simulink model "untitled"  (R2023a)
settings: Solver=VariableStepAuto  StartTime=0.0  StopTime=100  RelTol=1e-3
settings Model: Creator=Sumeadh  LastModifiedBy=Sumeadh

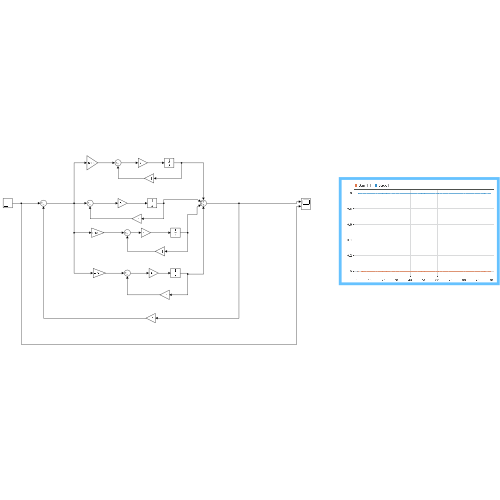
[thumbnail: Simulink's stored preview of the top-level diagram]
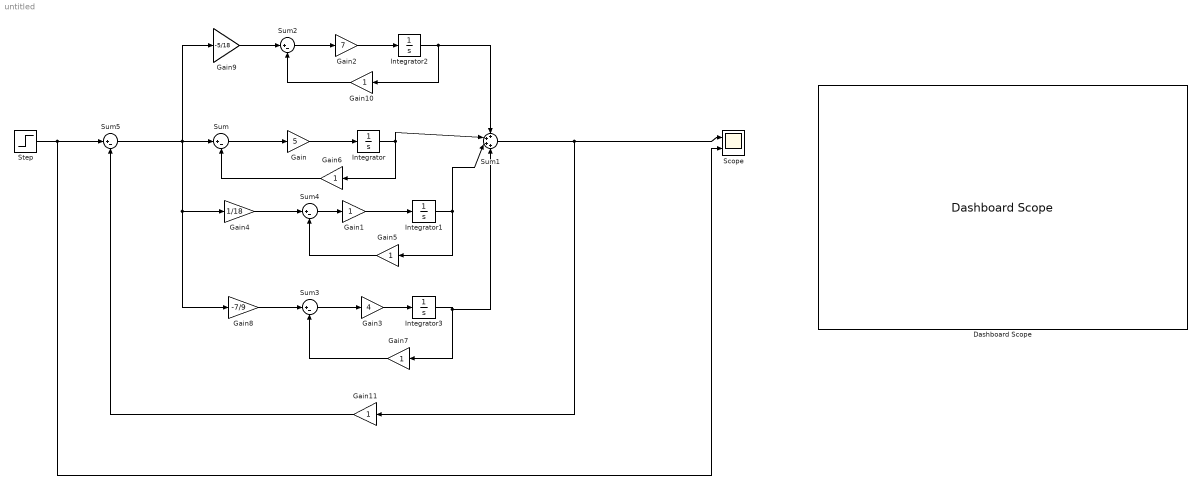
== system untitled ==
  Dashboard Scope : DashboardScope
  Gain : Gain  Gain=5
  Gain{1,5..7,10..11} (6 alike) : Gain
  Gain2 : Gain  Gain=7
  Gain3 : Gain  Gain=4
  Gain4 : Gain  Gain=1/18
  Gain8 : Gain  Gain=-7/9
  Gain9 : Gain  Gain=-5/18
  Integrator{,1..3} (4 alike) : Integrator
  Scope : Scope  NumInputPorts=2
  Step : Step  SampleTime=0
  Sum{,2..5} (5 alike) : Sum  Inputs=|+-
  Sum1 : Sum  Inputs=++++
  wires:
  Sum5/1 -> Gain9/1, Gain4/1, Gain8/1, Sum/1
  Sum/1 -> Gain/1
  Gain/1 -> Integrator/1
  Integrator/1 -> Sum1/2, Gain6/1
  Gain1/1 -> Integrator1/1
  Sum4/1 -> Gain1/1
  Integrator1/1 -> Sum1/3, Gain5/1
  Gain5/1 -> Sum4/2
  Gain4/1 -> Sum4/1
  Gain6/1 -> Sum/2
  Sum1/1 -> Gain11/1, Scope/1
  Gain3/1 -> Integrator3/1
  Integrator3/1 -> Sum1/4, Gain7/1
  Gain7/1 -> Sum3/2
  Sum3/1 -> Gain3/1
  Gain8/1 -> Sum3/1
  Sum2/1 -> Gain2/1
  Gain2/1 -> Integrator2/1
  Integrator2/1 -> Gain10/1, Sum1/1
  Gain10/1 -> Sum2/2
  Gain9/1 -> Sum2/1
  Step/1 -> Scope/2, Sum5/1
  Gain11/1 -> Sum5/2
